simulink model "lista2_lorenzslx"  (R2022b)
settings: Solver=FixedStepAuto  StartTime=0.0  StopTime=25.0  FixedStep=0.001  RelTol=1e-3
settings Model: Creator=mateu  LastModifiedBy=mateu

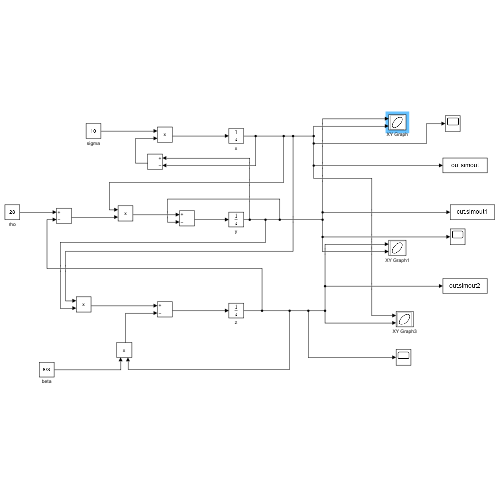
[thumbnail: Simulink's stored preview of the top-level diagram]
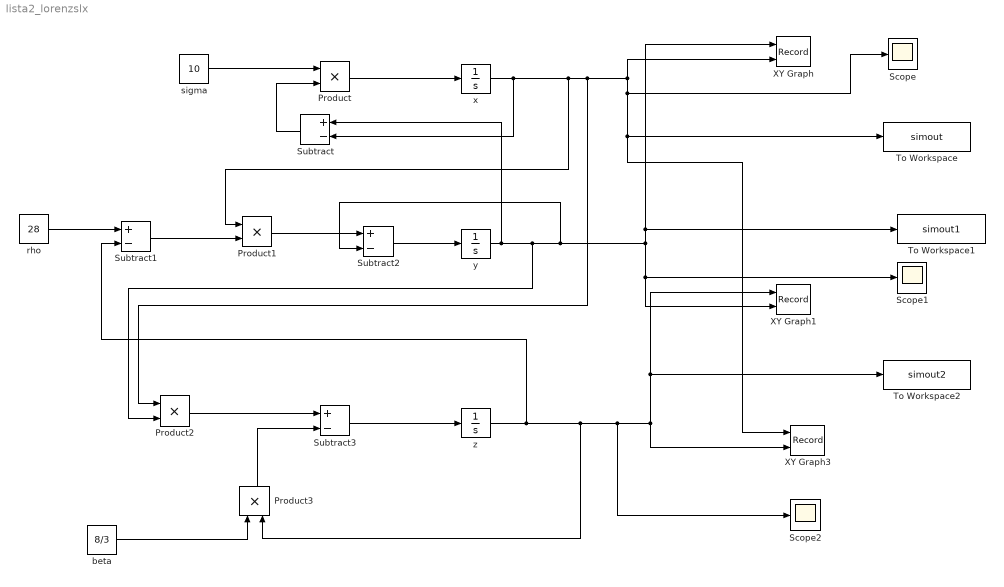
== system lista2_lorenzslx ==
  Product{,1..3} (4 alike) : Product
  Scope : Scope
  Scope1 : Scope
  Scope2 : Scope
  Subtract{,1..3} (4 alike) : Sum  Inputs=+-
  To Workspace : ToWorkspace  VariableName=simout  SampleTime=-1
  To Workspace1 : ToWorkspace  VariableName=simout1  SampleTime=-1
  To Workspace2 : ToWorkspace  VariableName=simout2  SampleTime=-1
  XY Graph : Record  FileSettingsInternal="{\"entries\":[{\"content\":{\"excelSettings\":{\"content\":{},\"type\":\"Streamout.ExcelSettings\"}},\"type\":\"Streamout.FileSettingStorage\",\"uuid\":\"13992367-6df8-4872-bd32-34eabf95292b\"}],\"packageUris\":[\"http://schema.mathworks.com/mf0/streamout_blocks/R2020a\"],\"version\":\"1.0\"}"  Layout=[1 1]  SignalsInternal="{\"entries\":[{\"content\":{\"signals\":[{\"content\":{\"blockPath\":[\"lista2_lorenzslx/XY Graph\"],\"channel\":[],\"dimensions\":[1],\"domain\":\"lista2_lorenzslx/XY Graph\",\"lineColor\":\"#a2142f\",\"plots\":[1],\"port\":1,\"sid\":[\"\"],\"signalID\":964,\"signalName\":\"y\"},\"type\":\"RecordBlkView.Signal\",\"uuid\":\"b91385a9-bdab-431e-ae58-12bcd1510d2c\"},{\"content\":{\"blockPath\":[\"lista2_lorenzslx/XY Graph\"],\"channel\":[],\"dimensions\":[1],\"domain\":\"lista2_lorenzslx/XY Graph\",\"lineColor\":\"#139fff\",\"plots\":[1],\"port\":2,\"sid\":[\"\"],\"signalID\":968,\"signalName\":\"x\"},\"type\":\"RecordBlkView.Signal\",\"uuid\":\"6d08cd55-e130-4c63-9ca9-5f07ea856c8a\"}]},\"type\":\"RecordBlkView.InputSignals\",\"uuid\":\"f4e593e5-a04d-448c-8125-55322691a080\"}],\"packageUris\":[\"http://schema.mathworks.com/mf0/streamout_blocks/R2020a\"],\"version\":\"1.0\"}"  VisualizationBindings="{\"xyplotplugin\":{\"info\":[{\"series\":[{\"bindingParametersList\":[{\"parameter\":\"X-Axis\",\"signalID\":964,\"signalName\":\"y\"},{\"parameter\":\"Y-Axis\",\"signalID\":968,\"signalName\":\"x\"}],\"seriesID\":43538}],\"subplotID\":1}]}}"  CompatibilityTag=XY
  XY Graph1 : Record  FileSettingsInternal="{\"entries\":[{\"content\":{\"excelSettings\":{\"content\":{},\"type\":\"Streamout.ExcelSettings\"}},\"type\":\"Streamout.FileSettingStorage\",\"uuid\":\"a5b5386f-6187-4de5-89fa-c94a53f00e27\"}],\"packageUris\":[\"http://schema.mathworks.com/mf0/streamout_blocks/R2020a\"],\"version\":\"1.0\"}"  Layout=[1 1]  SignalsInternal="{\"entries\":[{\"content\":{\"signals\":[{\"content\":{\"blockPath\":[\"lista2_lorenzslx/XY Graph1\"],\"channel\":[],\"dimensions\":[1],\"domain\":\"lista2_lorenzslx/XY Graph1\",\"lineColor\":\"#a2142f\",\"plots\":[1],\"port\":1,\"sid\":[\"\"],\"signalID\":972,\"signalName\":\"z\"},\"type\":\"RecordBlkView.Signal\",\"uuid\":\"de59c627-7218-433f-81bb-eecf63fc6559\"},{\"content\":{\"blockPath\":[\"lista2_lorenzslx/XY Graph1\"],\"channel\":[],\"dimensions\":[1],\"domain\":\"lista2_lorenzslx/XY Graph1\",\"lineColor\":\"#139fff\",\"plots\":[1],\"port\":2,\"sid\":[\"\"],\"signalID\":976,\"signalName\":\"y\"},\"type\":\"RecordBlkView.Signal\",\"uuid\":\"5a14de63-c6fd-4734-956c-2b683baa62bf\"}]},\"type\":\"RecordBlkView.InputSignals\",\"uuid\":\"3b2db215-7059-4689-913b-872ac8d4d864\"}],\"packageUris\":[\"http://schema.mathworks.com/mf0/streamout_blocks/R2020a\"],\"version\":\"1.0\"}"  VisualizationBindings="{\"xyplotplugin\":{\"info\":[{\"series\":[{\"bindingParametersList\":[{\"parameter\":\"X-Axis\",\"signalID\":972,\"signalName\":\"z\"},{\"parameter\":\"Y-Axis\",\"signalID\":976,\"signalName\":\"y\"}],\"seriesID\":10459}],\"subplotID\":1}]}}"  CompatibilityTag=XY
  XY Graph3 : Record  FileSettingsInternal="{\"entries\":[{\"content\":{\"excelSettings\":{\"content\":{},\"type\":\"Streamout.ExcelSettings\"}},\"type\":\"Streamout.FileSettingStorage\",\"uuid\":\"8b067cb2-b9e7-4c6e-a722-a4a4f1857175\"}],\"packageUris\":[\"http://schema.mathworks.com/mf0/streamout_blocks/R2020a\"],\"version\":\"1.0\"}"  Layout=[1 1]  SignalsInternal="{\"entries\":[{\"content\":{\"signals\":[{\"content\":{\"blockPath\":[\"lista2_lorenzslx/XY Graph3\"],\"channel\":[],\"dimensions\":[1],\"domain\":\"lista2_lorenzslx/XY Graph3\",\"lineColor\":\"#a2142f\",\"plots\":[1],\"port\":1,\"sid\":[\"\"],\"signalID\":980,\"signalName\":\"x\"},\"type\":\"RecordBlkView.Signal\",\"uuid\":\"73cc697e-a626-4313-bea3-9904ef05703f\"},{\"content\":{\"blockPath\":[\"lista2_lorenzslx/XY Graph3\"],\"channel\":[],\"dimensions\":[1],\"domain\":\"lista2_lorenzslx/XY Graph3\",\"lineColor\":\"#139fff\",\"plots\":[1],\"port\":2,\"sid\":[\"\"],\"signalID\":984,\"signalName\":\"z\"},\"type\":\"RecordBlkView.Signal\",\"uuid\":\"1e38e6aa-1bba-4421-8fdf-11dbb0298e48\"}]},\"type\":\"RecordBlkView.InputSignals\",\"uuid\":\"b8c13616-d123-4f69-be45-795cd6958a71\"}],\"packageUris\":[\"http://schema.mathworks.com/mf0/streamout_blocks/R2020a\"],\"version\":\"1.0\"}"  VisualizationBindings="{\"xyplotplugin\":{\"info\":[{\"series\":[{\"bindingParametersList\":[{\"parameter\":\"X-Axis\",\"signalID\":980,\"signalName\":\"x\"},{\"parameter\":\"Y-Axis\",\"signalID\":984,\"signalName\":\"z\"}],\"seriesID\":2059}],\"subplotID\":1}]}}"  CompatibilityTag=XY
  beta : Constant  Value=8/3
  rho : Constant  Value=28
  sigma : Constant  Value=10
  x : Integrator  InitialCondition=1
  y : Integrator  InitialCondition=1
  z : Integrator  InitialCondition=1
  wires:
  y/1 -> Product2/2, Subtract2/2, Scope1/1, XY Graph1/2, XY Graph/1, To Workspace1/1, Subtract/1
  x/1 -> Product1/1, Product2/1, Scope/1, XY Graph3/1, To Workspace/1, XY Graph/2, Subtract/2
  z/1 -> Subtract1/2, Product3/2, Scope2/1, XY Graph3/2, To Workspace2/1, XY Graph1/1
  Subtract/1 -> Product/2
  Product/1 -> x/1
  sigma/1 -> Product/1
  rho/1 -> Subtract1/1
  Subtract1/1 -> Product1/2
  Product1/1 -> Subtract2/1
  Subtract2/1 -> y/1
  Subtract3/1 -> z/1
  Product2/1 -> Subtract3/1
  Product3/1 -> Subtract3/2
  beta/1 -> Product3/1
